simulink model "priority"  (R2022a)
settings: Solver=VariableStepAuto  StartTime=0.0  StopTime=10.0  RelTol=1e-3
undefined symbols (not defined in the file or in its folder): A1, A2, A3, B1, B2, B3
libraries: truetime x4
settings Model: Creator=vishn  LastModifiedBy=vishn

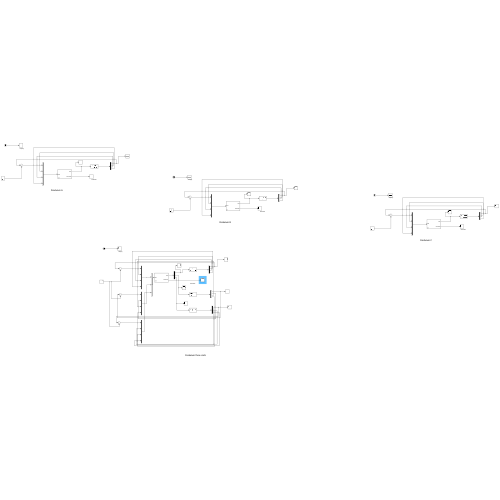
[thumbnail: Simulink's stored preview of the top-level diagram]
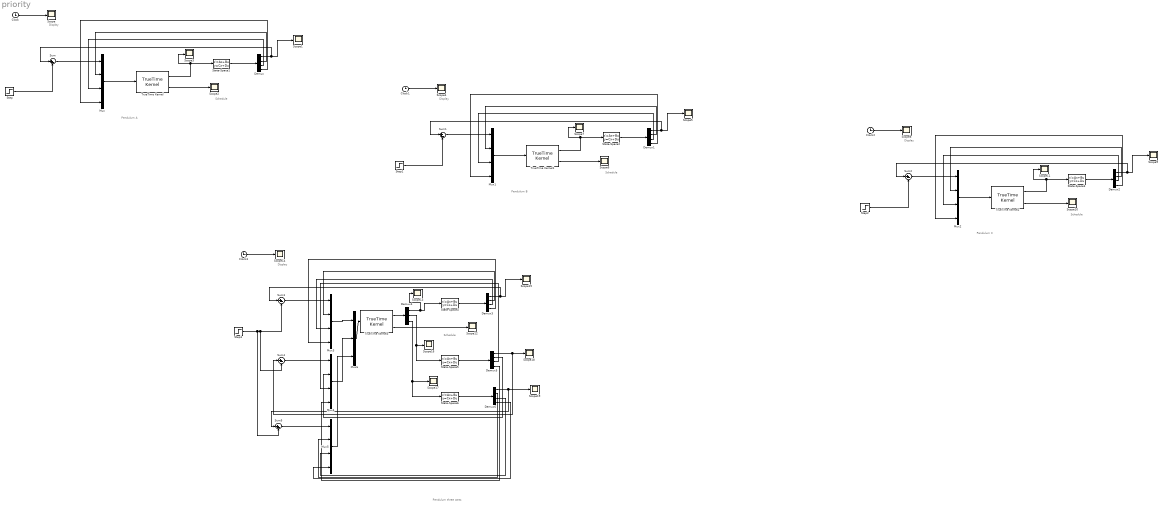
== system priority ==
  note: Pendulum A
  note: Schedule
  note: Display
  note: Pendulum B
  note: Schedule
  note: Display
  note: Schedule
  note: Pendulum C
  note: Display
  note: Pendulum three carts
  note: Display
  note: Schedule
  Clock{,1..3} (4 alike) : Clock
  Demux{,1..3,5..6} (6 alike) : Demux
  Demux4 : Demux  Outputs=3
  Mux{,1..5} (6 alike) : Mux
  Mux6 : Mux  Inputs=3
  Scope{,1..19} (20 alike) : Scope
  State-Space1 : StateSpace  A=A1  B=B1  C=eye(4)  D=zeros(4,1)  InitialCondition=[0;0;0;0]
  State-Space2 : StateSpace  A=A3  B=B3  C=eye(4)  D=zeros(4,1)  InitialCondition=[0;0;0;0]
  State-Space3 : StateSpace  A=A2  B=B2  C=eye(4)  D=zeros(4,1)  InitialCondition=[0;0;0;0]
  State-Space4 : StateSpace  A=A1  B=B1  C=eye(4)  D=zeros(4,1)  InitialCondition=[0;0;0;0]
  State-Space5 : StateSpace  A=A2  B=B2  C=eye(4)  D=zeros(4,1)  InitialCondition=[0;0;0;0]
  State-Space6 : StateSpace  A=A3  B=B3  C=eye(4)  D=zeros(4,1)  InitialCondition=[0;0;0;0]
  Step{,1..3} (4 alike) : Step  SampleTime=0
  Sum{,1..5} (6 alike) : Sum  Inputs=|+-
  TrueTime Kernel : truetime/TrueTime Kernel  sfun=node_init  args=1  ninputsoutputs=[4 1]  ntriggers=0  trigtype=falling  nwnodenbr=[]  clockoffsetdrift=[0 0]  schedoutput=on  battery=off  poweroutput=off
  TrueTime Kernel1 : truetime/TrueTime Kernel  sfun=node_initB  args=1  ninputsoutputs=[4 1]  ntriggers=0  trigtype=falling  nwnodenbr=[]  clockoffsetdrift=[0 0]  schedoutput=on  battery=off  poweroutput=off
  TrueTime Kernel2 : truetime/TrueTime Kernel  sfun=node_initC  args=1  ninputsoutputs=[4 1]  ntriggers=0  trigtype=falling  nwnodenbr=[]  clockoffsetdrift=[0 0]  schedoutput=on  battery=off  poweroutput=off
  TrueTime Kernel3 : truetime/TrueTime Kernel  sfun=node_init_three_carts  args=1  ninputsoutputs=[12 3]  ntriggers=0  trigtype=falling  nwnodenbr=[]  clockoffsetdrift=[0 0]  schedoutput=on  battery=off  poweroutput=off
  wires:
  Clock/1 -> Scope/1
  Step/1 -> Sum/2
  Sum/1 -> Mux/1
  State-Space1/1 -> Demux/1
  Mux/1 -> TrueTime Kernel/1
  Demux/1 -> Sum/1, Scope1/1
  Demux/2 -> Mux/2
  Demux/3 -> Mux/3
  Demux/4 -> Mux/4
  TrueTime Kernel/2 -> Scope2/1
  TrueTime Kernel/1 -> Scope3/1, State-Space1/1
  Demux1/3 -> Mux1/3
  Demux1/4 -> Mux1/4
  TrueTime Kernel1/2 -> Scope6/1
  Sum1/1 -> Mux1/1
  Demux1/1 -> Sum1/1, Scope5/1
  Step1/1 -> Sum1/2
  Mux1/1 -> TrueTime Kernel1/1
  Demux1/2 -> Mux1/2
  State-Space2/1 -> Demux1/1
  Clock1/1 -> Scope4/1
  TrueTime Kernel1/1 -> Scope7/1, State-Space2/1
  Demux2/3 -> Mux2/3
  Clock2/1 -> Scope8/1
  State-Space3/1 -> Demux2/1
  TrueTime Kernel2/1 -> Scope11/1, State-Space3/1
  TrueTime Kernel2/2 -> Scope10/1
  Sum2/1 -> Mux2/1
  Mux2/1 -> TrueTime Kernel2/1
  Step2/1 -> Sum2/2
  Demux2/4 -> Mux2/4
  Demux2/1 -> Sum2/1, Scope9/1
  Demux2/2 -> Mux2/2
  Demux3/4 -> Mux3/4
  Sum3/1 -> Mux3/1
  Demux3/2 -> Mux3/2
  TrueTime Kernel3/2 -> Scope12/1
  Demux3/1 -> Sum3/1, Scope15/1
  Demux3/3 -> Mux3/3
  State-Space4/1 -> Demux3/1
  Step3/1 -> Sum5/2, Sum4/2, Sum3/2
  Clock3/1 -> Scope14/1
  Mux3/1 -> Mux6/1
  Mux4/1 -> Mux6/2
  Mux5/1 -> Mux6/3
  Mux6/1 -> TrueTime Kernel3/1
  Sum4/1 -> Mux4/1
  Sum5/1 -> Mux5/1
  TrueTime Kernel3/1 -> Demux4/1
  Demux4/1 -> Scope13/1, State-Space4/1
  Demux4/2 -> State-Space5/1, Scope16/1
  Demux4/3 -> Scope17/1, State-Space6/1
  State-Space5/1 -> Demux5/1
  State-Space6/1 -> Demux6/1
  Demux6/1 -> Sum5/1, Scope19/1
  Demux5/1 -> Sum4/1, Scope18/1
  Demux5/2 -> Mux4/2
  Demux5/3 -> Mux4/3
  Demux5/4 -> Mux4/4
  Demux6/2 -> Mux5/2
  Demux6/3 -> Mux5/3
  Demux6/4 -> Mux5/4
